simulink model "task2simulink"  (R2016a)
settings: Solver=VariableStepAuto  StartTime=0.0  StopTime=10.0  RelTol=1e-3
libraries: dspsrcs4 x1
settings Model: Creator=admin  LastModifiedBy=admin

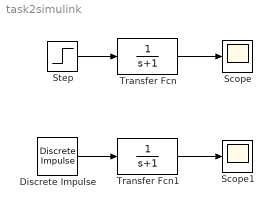
== system task2simulink ==
  Discrete Impulse : dspsrcs4/Discrete  Impulse  Delay=0  SampleTime=0.001  FrameSample=1  OutputFrames=off  dataType=double  isSigned=on  wordLen=16  udDataType=sfix(16)  fracBitsMode=Best precision  numFracBits=15  OutDataTypeStr=double  LastOutDataTypeStr=double
  Scope : Scope
  Scope1 : Scope
  Step : Step  Time=0  Before=1  SampleTime=0
  Transfer Fcn : TransferFcn  Denominator=[1 1]
  Transfer Fcn1 : TransferFcn  Denominator=[1 1]
  wires:
  Step/1 -> Transfer Fcn/1
  Transfer Fcn/1 -> Scope/1
  Discrete Impulse/1 -> Transfer Fcn1/1
  Transfer Fcn1/1 -> Scope1/1
